simulink model "MachineThree_2022a"  (R2022a)
settings: Solver=FixedStepAuto  StartTime=0.0  StopTime=inf  RelTol=1e-3  EnableMultiTasking=on
libraries: arduinolib x2
settings Model: ExtModeTrigDuration=2  Creator=nikhi  LastModifiedBy=Lagadh Matsa
settings SolverCC: AlgebraicLoopSolver=TrustRegion
settings OptimizationCC: EnhancedBackFolding=on  PassReuseOutputArgsThreshold=0  MaxStackSize=64  OptimizeBlockOrder=speed  DifferentSizesBufferReuse=on  OptimizationCustomize=off
settings DebuggingCC: ParameterTunabilityLossMsg=error  UnconnectedInputMsg=warning  UnconnectedOutputMsg=warning  UnconnectedLineMsg=warning  SFMachineParentedDataDiag=warning
settings HardwareCC: ProdBitPerInt=16  ProdBitPerPointer=16  ProdBitPerSizeT=16  ProdBitPerPtrDiffT=16  ProdLargestAtomicFloat=None  ProdWordSize=8  ProdHWDeviceType=Atmel->AVR  UseEmbeddedCoderFeatures=off  UseSimulinkCoderFeatures=off
settings SFSimCC: MATLABDynamicMemAlloc=off
settings RTWCC: SystemTargetFile=ert.tlc  HardwareBoard=Arduino Uno  TemplateMakefile=ert_default_tmf  Toolchain=Arduino AVR  BuildConfiguration=Faster Runs  DLArmComputeVersion=19.05
settings CodeAppCC: ForceParamTrailComments=on  OperatorAnnotations=on
settings ERTTargetCC: ERTCustomFileBanners=off  SupportContinuousTime=on  SupportNonInlinedSFcns=on  RemoveResetFunc=off  SupportVariableSizeSignals=on  ModelStepFunctionPrototypeControlCompliant=off  ExtModeStaticAllocSize=250

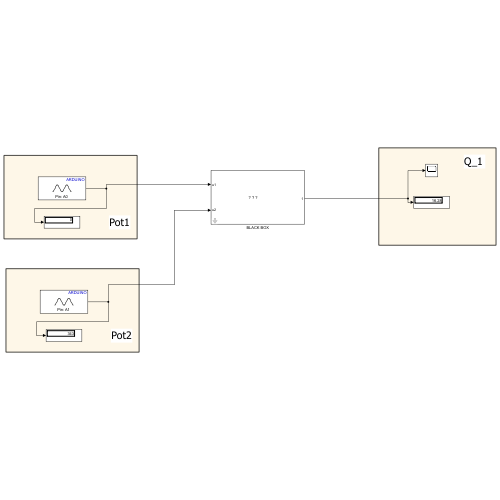
[thumbnail: Simulink's stored preview of the top-level diagram]
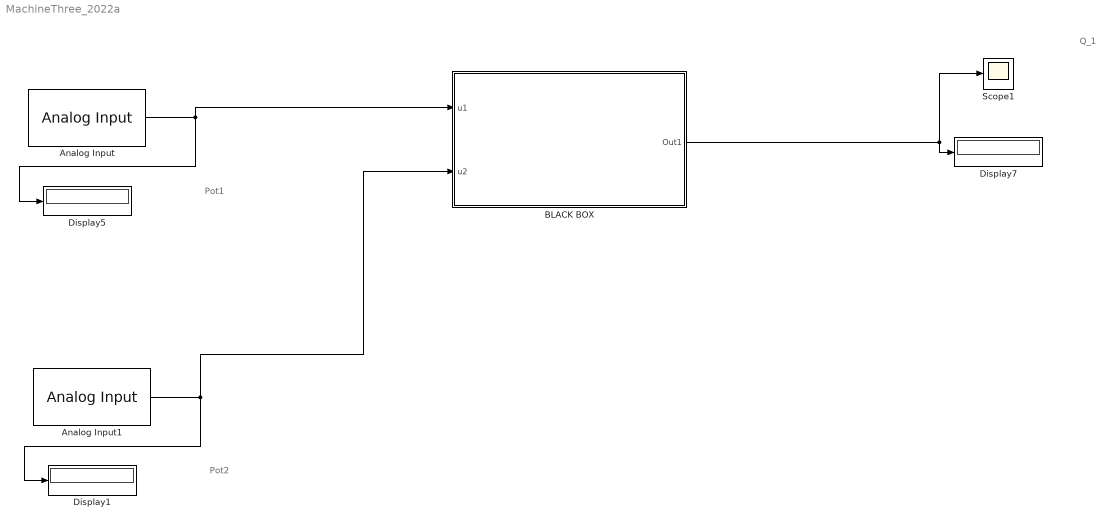
== system MachineThree_2022a ==
  note: Q_1
  note: Pot1
  note: Pot2
  Analog Input : arduinolib/Analog Input  pinNumber=0  ReadResultsOnly=off  ConversionTriggerSource=Software  ExternalTriggerType=uint32( 0 )  OutputDataType=uint16  EnableConversionCompleteNotify=off  EnableOuputStatus=off  SampleTime=1  blockPlatform=arduino
  Analog Input1 : arduinolib/Analog Input  pinNumber=1  ReadResultsOnly=off  ConversionTriggerSource=Software  ExternalTriggerType=uint32( 0 )  OutputDataType=uint16  EnableConversionCompleteNotify=off  EnableOuputStatus=off  SampleTime=1  blockPlatform=arduino
  BLACK BOX : Subsystem
      mask Display: image('1.jfif'); % Use "Edit Image" on toolstrip to change.
  Display1 : Display
  Display5 : Display
  Display7 : Display
  Scope1 : Scope
  wires:
  Analog Input/1 -> Display5/1, BLACK BOX/1(u1)
  BLACK BOX/1(Out1) -> Scope1/1, Display7/1
  Analog Input1/1 -> BLACK BOX/2(u2), Display1/1

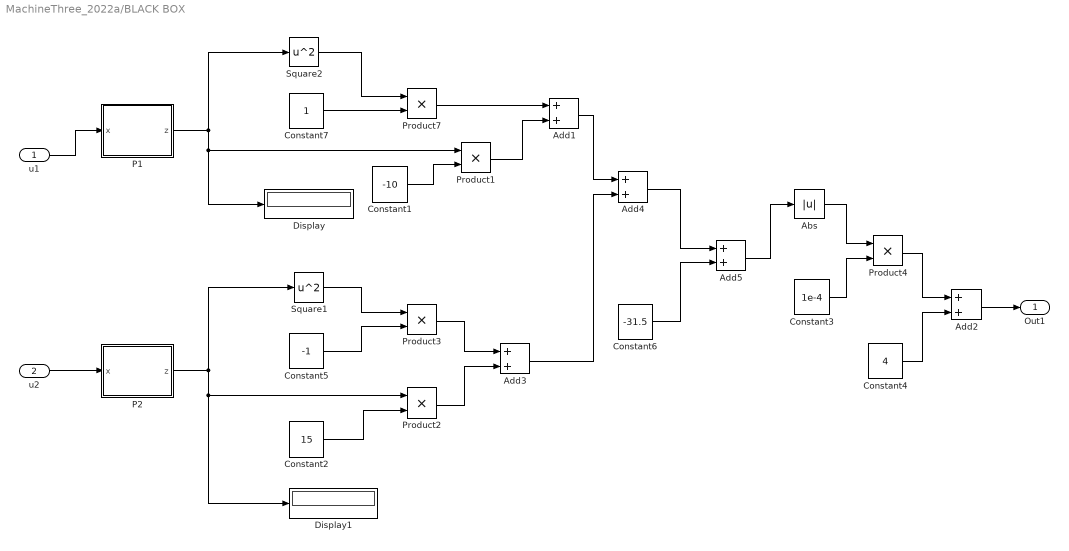
== system MachineThree_2022a/BLACK BOX ==
  u1 : Inport
  u2 : Inport  Port=2
  Abs : Abs  SaturateOnIntegerOverflow=off
  Add{1..5} (5 alike) : Sum
  Constant1 : Constant  Value=-10
  Constant2 : Constant  Value=15
  Constant3 : Constant  Value=1e-4
  Constant4 : Constant  Value=4
  Constant5 : Constant  Value=-1
  Constant6 : Constant  Value=-31.5
  Constant7 : Constant
  Display : Display
  Display1 : Display
  P1 : MATLAB Function  TreatAsAtomicUnit=on
  P2 : MATLAB Function  TreatAsAtomicUnit=on
  Product{1..4,7} (5 alike) : Product
  Square1 : Math  Operator=square
  Square2 : Math  Operator=square
  Out1 : Outport
  wires:
  Constant7/1 -> Product7/2
  P1/1(z) -> Display/1, Product1/1, Square2/1
  u1/1 -> P1/1(x)
  Square2/1 -> Product7/1
  P2/1(z) -> Display1/1, Product2/1, Square1/1
  Constant5/1 -> Product3/2
  u2/1 -> P2/1(x)
  Square1/1 -> Product3/1
  Constant1/1 -> Product1/2
  Product7/1 -> Add1/1
  Product1/1 -> Add1/2
  Constant2/1 -> Product2/2
  Abs/1 -> Product4/1
  Constant3/1 -> Product4/2
  Product4/1 -> Add2/1
  Constant4/1 -> Add2/2
  Add2/1 -> Out1/1
  Product3/1 -> Add3/1
  Product2/1 -> Add3/2
  Add1/1 -> Add4/1
  Add3/1 -> Add4/2
  Constant6/1 -> Add5/2
  Add4/1 -> Add5/1
  Add5/1 -> Abs/1

== matlab function MachineThree_2022a/BLACK BOX/P1 ==
  data: x input; z output
function z = fcn(x)
z = 0;
if x < 512
    z = (double(x)*-1);
else
    z = double(x)*0.5;
end
z = z;

== matlab function MachineThree_2022a/BLACK BOX/P2 ==
  data: x input; z output
function z = fcn(x)
z = 0;
if x < 512
    z = (double(x)*-1);
else
    z = double(x)*0.5;
end
z = z;
